simulink model "stabilizer"  (R2017a)
settings: Solver=VariableStepAuto  StartTime=0.0  StopTime=inf  RelTol=1e-3
settings Model: Creator=mini  LastModifiedBy=mini

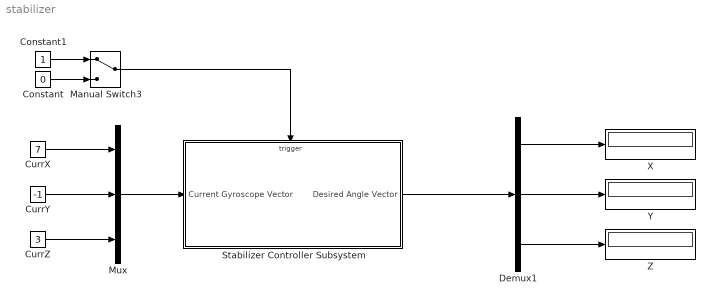
== system stabilizer ==
  Constant : Constant  Value=0
  Constant1 : Constant
  CurrX : Constant  Value=7
  CurrY : Constant  Value=-1
  CurrZ : Constant  Value=3
  Demux1 : Demux  Outputs=3
  Manual Switch3 : ManualSwitch
  Mux : Mux  Inputs=3
  Stabilizer Controller Subsystem : Subsystem
  X : Display
  Y : Display
  Z : Display
  wires:
  Demux1/3 -> Z/1
  Manual Switch3/1 -> Stabilizer Controller Subsystem/Trigger
  Demux1/2 -> Y/1
  Constant/1 -> Manual Switch3/2
  Constant1/1 -> Manual Switch3/1
  Stabilizer Controller Subsystem/1(Desired Angle Vector) -> Demux1/1
  Demux1/1 -> X/1
  Mux/1 -> Stabilizer Controller Subsystem/1(Current Gyroscope Vector)
  CurrX/1 -> Mux/1
  CurrY/1 -> Mux/2
  CurrZ/1 -> Mux/3

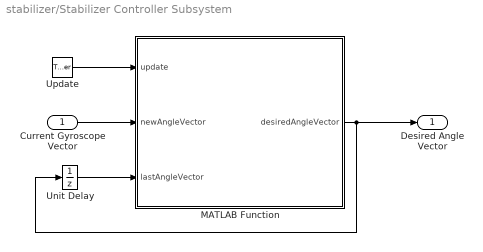
== system stabilizer/Stabilizer Controller Subsystem ==
  Current Gyroscope Vector : Inport
  Update : TriggerPort  VariantControl=Variant  ShowOutputPort=on  PortDimensions=1
  MATLAB Function : MATLAB Function  TreatAsAtomicUnit=on
  Unit Delay : UnitDelay  SampleTime=-1
  Desired Angle Vector : Outport
  wires:
  Unit Delay/1 -> MATLAB Function/3(lastAngleVector)
  MATLAB Function/1(desiredAngleVector) -> Desired Angle Vector/1, Unit Delay/1
  Update/1 -> MATLAB Function/1(update)
  Current Gyroscope Vector/1 -> MATLAB Function/2(newAngleVector)

== matlab function stabilizer/Stabilizer Controller Subsystem/MATLAB Function ==
  data: update input; newAngleVector input; desiredAngleVector output; lastAngleVector input
function desiredAngleVector = fcn(update, newAngleVector, lastAngleVector)
    % default action on startup 
    if ( update )
        desiredAngleVector = newAngleVector;
    else
        desiredAngleVector = lastAngleVector;
    end
